simulink model "three_level_svpwm"  (R2013a)
settings: Solver=ode45  StartTime=0.0  StopTime=1  MaxStep=1e-3  RelTol=1e-3
libraries: powerlib x13, simulink x8, commutil2 x4, powerlib_meascontrol x3
settings Model: Creator=HXXXIA001  LastModifiedBy=HXXXIA001

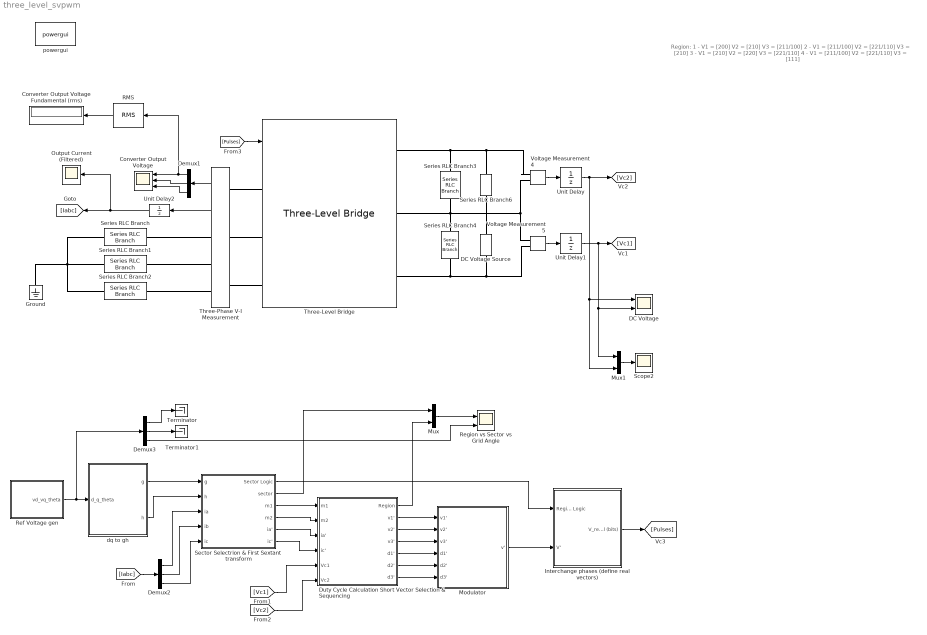
== system three_level_svpwm ==
  note: Region:
      | 1 - V1 = [200]	   V2 = [210]   V3 = [211/100]
      | 2 - V1 = [211/100]   V2 = [221/110]   V3 = [210]
      | 3 - V1 = [210]   V2 = [220]   V3 = [221/110]
      | 4 - V1 = [211/100]   V2 = [221/110]   V3 = [111]
  Converter Output Voltage : Scope  NumInputPorts=3
      settings: YMin=-120~-120~-120  YMax=120~120~120  SaveName=Vph
  Converter Output Voltage Fundamental (rms) : Display
  DC Voltage : Scope  NumInputPorts=2
      settings: YMin=59.65~59.725  YMax=60.3~60.275
  DC Voltage Source : powerlib/Electrical Sources/DC Voltage Source  Amplitude=120  Measurements=None
  Demux1 : Demux  Outputs=3
  Demux2 : Demux  Outputs=3
  Demux3 : Demux  Outputs=3
  Duty Cycle Calculation Short Vector Selection & Sequencing : Subsystem
  Ground : powerlib/Elements/Ground  LConnTagsString=a
  Interchange phases (define real vectors) : Subsystem
  Modulator : Subsystem  mask{Tm=5e-5, Ts=5e-6}
      mask prompts: Tm "Converter Modulation Period (s)"; Ts "Clock Sampling Period (s)"
  Mux : Mux  Inputs=2
  Mux1 : Mux  Inputs=2
  Output Current (Filtered) : Scope
      settings: YMin=-80  YMax=80  SaveName=Iph
  RMS : powerlib_meascontrol/Measurements/RMS  TrueRMS=on  Freq=50  RMSInit=0  Ts=5e-5
  Ref Voltage gen : Subsystem  mask{m=0.8, f=50}
      mask prompts: m "Modulation Index ( 0<m<1 )"; f "Fundamental Frequency (Hz)"
  Region vs Sector vs Grid Angle : Scope  NumInputPorts=2
      settings: YMin=-5~-5  YMax=5~5  SaveName=ScopeData3
  Scope2 : Scope
      settings: SaveName=ScopeData2
  Sector Selectrion & First Sextant transform : Subsystem
  Series RLC Branch : powerlib/Elements/Series RLC Branch  LConnTagsString=__new0  RConnTagsString=__new0  BranchType=RL  Resistance=10  Inductance=4e-3  SetiL0=off  InitialCurrent=0  Capacitance=1e-6  Setx0=off  InitialVoltage=0  Measurements=None
  Series RLC Branch1 : powerlib/Elements/Series RLC Branch  LConnTagsString=__new0  RConnTagsString=__new0  BranchType=RL  Resistance=10  Inductance=4e-3  SetiL0=off  InitialCurrent=0  Capacitance=1e-6  Setx0=off  InitialVoltage=0  Measurements=None
  Series RLC Branch2 : powerlib/Elements/Series RLC Branch  LConnTagsString=__new0  RConnTagsString=__new0  BranchType=RL  Resistance=10  Inductance=4e-3  SetiL0=off  InitialCurrent=0  Capacitance=1e-6  Setx0=off  InitialVoltage=0  Measurements=None
  Series RLC Branch3 : powerlib/Elements/Series RLC Branch  LConnTagsString=__new0  RConnTagsString=__new0  BranchType=C  Resistance=0.0001  Inductance=1e-3  SetiL0=off  InitialCurrent=0  Capacitance=4700e-6  Setx0=on  InitialVoltage=60  Measurements=None
  Series RLC Branch4 : powerlib/Elements/Series RLC Branch  LConnTagsString=__new0  RConnTagsString=__new0  BranchType=C  Resistance=0.0001  Inductance=1e-3  SetiL0=off  InitialCurrent=0  Capacitance=4700e-6  Setx0=on  InitialVoltage=60  Measurements=None
  Series RLC Branch6 : powerlib/Elements/Series RLC Branch  LConnTagsString=__new0  RConnTagsString=__new0  BranchType=R  Resistance=1e-3  Inductance=1e-3  SetiL0=off  InitialCurrent=0  Capacitance=4700e-6  Setx0=off  InitialVoltage=0  Measurements=None
  Terminator : Terminator
  Terminator1 : Terminator
  Three-Level Bridge : powerlib/Power Electronics/Three-Level Bridge  Arms=3  SnubberResistance=1e5  SbubberCapacitance=inf  Device=IGBT / Diodes  Ron=1e-3  ForwardVoltages="[  0  0  ]"  Measurements=None
  Three-Phase V-I Measurement : powerlib/Measurements/Three-Phase V-I Measurement  VoltageMeasurement=phase-to-ground  SetLabelV=off  LabelV=Vabc  Vpu=off  VpuLL=off  CurrentMeasurement=yes  SetLabelI=off  LabelI=Iabc  Ipu=off  Pbase=100e6  Vbase=500e3  OutputType=Complex  PhasorSimulation=off  PSBequivalent=0
  Unit Delay : UnitDelay  SampleTime=-1
  Unit Delay1 : UnitDelay  SampleTime=-1
  Unit Delay2 : UnitDelay  SampleTime=-1
  Voltage Measurement4 : powerlib/Measurements/Voltage Measurement  PhasorSimulation=off  OutputType=Complex  PSBequivalent=0
  Voltage Measurement5 : powerlib/Measurements/Voltage Measurement  PhasorSimulation=off  OutputType=Complex  PSBequivalent=0
  dq to gh : Subsystem
  powergui : powerlib/powergui  Priority=1  SimulationMode=Discrete  SolverType=Tustin  SampleTime=5e-6  frequency=60  SPID=off  DisableSnubberDevices=off  DisableRonSwitches=off  DisableVfSwitches=off  SwTol=0  Interpol=off  DisplayEquations=off  frequencyindice=0  Pbase=100e6  ErrMax=1e-4  Iterations=50  UnitsV=kV  UnitsW=MW  FunctionMessages=off  echomessages=off  HookPort=off  EnableUseOfTLC=off  x0status=blocks  RestoreLinks=warning  ResistiveCurrentMeasurement=off  Frange=[0:2:500]  Ylog=off  Xlog=on  ShowGrid=off  save=off  variable=ZData  structure=Iph  ZoomFFT=off  StartTime=0.0  cycles=10  DisplayStyle=1  fundamental=50  FreqAxis=off  MaxFrequency=2000  frequencyindicesteady=1  RmsSteady=1  display=off  Ts=0  methode=off
  wires:
  Ref Voltage gen/1(vd_vq_theta) -> Demux3/1, dq to gh/1(d_q_theta)
  Sector Selectrion & First Sextant transform/3(m1) -> Duty Cycle Calculation Short Vector Selection & Sequencing/1(m1)
  Sector Selectrion & First Sextant transform/4(m2) -> Duty Cycle Calculation Short Vector Selection & Sequencing/2(m2)
  Sector Selectrion & First Sextant transform/2(sector) -> Mux/1
  Mux/1 -> Region vs Sector vs Grid Angle/1
  Duty Cycle Calculation Short Vector Selection & Sequencing/1(Region) -> Mux/2
  dq to gh/1(g) -> Sector Selectrion & First Sextant transform/1(g)
  dq to gh/2(h) -> Sector Selectrion & First Sextant transform/2(h)
  Sector Selectrion & First Sextant transform/5(ia') -> Duty Cycle Calculation Short Vector Selection & Sequencing/3(ia')
  Sector Selectrion & First Sextant transform/6(ic') -> Duty Cycle Calculation Short Vector Selection & Sequencing/4(ic')
  Duty Cycle Calculation Short Vector Selection & Sequencing/2(v1') -> Modulator/1(v1')
  Duty Cycle Calculation Short Vector Selection & Sequencing/3(v2') -> Modulator/2(v2')
  Duty Cycle Calculation Short Vector Selection & Sequencing/4(v3') -> Modulator/3(v3')
  Duty Cycle Calculation Short Vector Selection & Sequencing/5(d1') -> Modulator/4(d1')
  Duty Cycle Calculation Short Vector Selection & Sequencing/6(d2') -> Modulator/5(d2')
  Duty Cycle Calculation Short Vector Selection & Sequencing/7(d3') -> Modulator/6(d3')
  Sector Selectrion & First Sextant transform/1(Sector Logic) -> Interchange phases (define real vectors)/1(Region Logic)
  Modulator/1(v') -> Interchange phases (define real vectors)/2(V')
  Three-Phase V-I Measurement/1 -> Demux1/1
  Demux1/1 -> Converter Output Voltage/1, RMS/1
  Demux1/2 -> Converter Output Voltage/2
  Demux1/3 -> Converter Output Voltage/3
  Voltage Measurement4/1 -> Unit Delay/1
  Unit Delay/1 -> Mux1/2, DC Voltage/1, [Vc2]
  Voltage Measurement5/1 -> Unit Delay1/1
  Unit Delay1/1 -> Mux1/1, DC Voltage/2, [Vc1]
  [Iabc] -> Demux2/1
  Demux2/1 -> Sector Selectrion & First Sextant transform/3(ia)
  Demux2/2 -> Sector Selectrion & First Sextant transform/4(ib)
  Demux2/3 -> Sector Selectrion & First Sextant transform/5(ic)
  [Vc1] -> Duty Cycle Calculation Short Vector Selection & Sequencing/5(Vc1)
  [Vc2] -> Duty Cycle Calculation Short Vector Selection & Sequencing/6(Vc2)
  Three-Phase V-I Measurement/2 -> Unit Delay2/1
  Unit Delay2/1 -> Output Current (Filtered)/1, [Iabc]
  Mux1/1 -> Scope2/1
  RMS/1 -> Converter Output Voltage Fundamental (rms)/1
  Demux3/1 -> Terminator/1
  Demux3/2 -> Terminator1/1
  Demux3/3 -> Region vs Sector vs Grid Angle/2
  Interchange phases (define real vectors)/1(V_real (bits)) -> [Pulses]
  [Pulses] -> Three-Level Bridge/1
  connections:
  Voltage Measurement4/LConn1 -- Series RLC Branch6/LConn1 -- Three-Level Bridge/RConn1 -- Series RLC Branch3/LConn1
  Voltage Measurement5/LConn2 -- Three-Level Bridge/RConn3 -- Series RLC Branch4/RConn1 -- DC Voltage Source/LConn1
  Series RLC Branch/RConn1 -- Ground/LConn1 -- Series RLC Branch2/RConn1 -- Series RLC Branch1/RConn1
  Three-Phase V-I Measurement/LConn1 -- Three-Level Bridge/LConn1
  Three-Phase V-I Measurement/LConn2 -- Three-Level Bridge/LConn2
  Three-Phase V-I Measurement/LConn3 -- Three-Level Bridge/LConn3
  Series RLC Branch/LConn1 -- Three-Phase V-I Measurement/RConn1
  Series RLC Branch1/LConn1 -- Three-Phase V-I Measurement/RConn2
  Series RLC Branch2/LConn1 -- Three-Phase V-I Measurement/RConn3
  Voltage Measurement4/LConn2 -- Three-Level Bridge/RConn2 -- Series RLC Branch4/LConn1 -- Series RLC Branch3/RConn1 -- Voltage Measurement5/LConn1
  Series RLC Branch6/RConn1 -- DC Voltage Source/RConn1

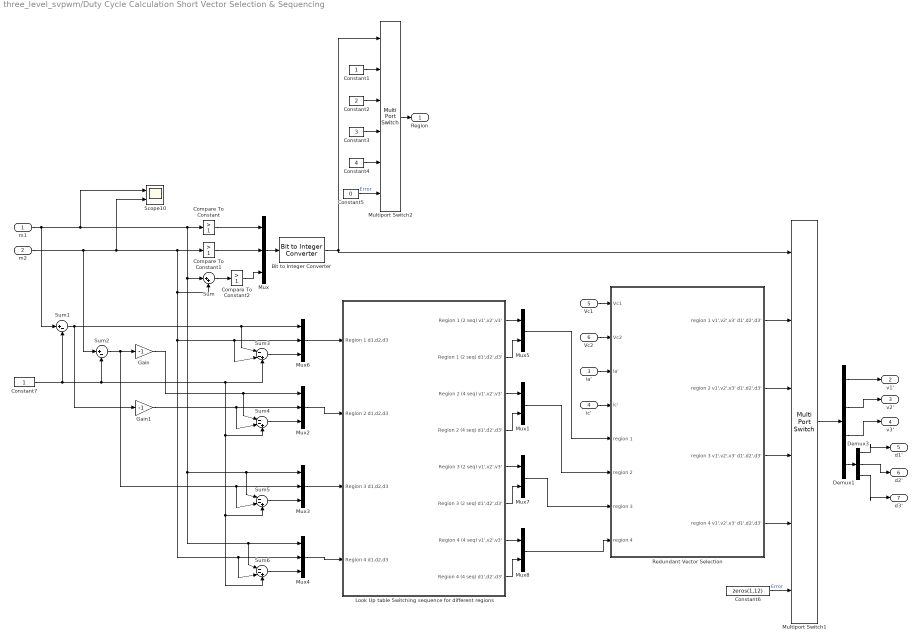
== system three_level_svpwm/Duty Cycle Calculation Short Vector Selection & Sequencing ==
  m1 : Inport
  m2 : Inport  Port=2
  ia' : Inport  Port=3
  ic' : Inport  Port=4
  Vc1 : Inport  Port=5
  Vc2 : Inport  Port=6
  Bit to Integer Converter : commutil2/Bit to Integer Converter  nbits=3  bitOrder=MSB first  signedOutputValues=Unsigned  outDtype=Inherit via internal rule  outDtypeSigned=Inherit via internal rule
  Compare To Constant : simulink/Logic and Bit Operations/Compare To Constant  relop=>  const=1  OutDataTypeStr=boolean
  Compare To Constant1 : simulink/Logic and Bit Operations/Compare To Constant  relop=>  const=1  OutDataTypeStr=boolean
  Compare To Constant2 : simulink/Logic and Bit Operations/Compare To Constant  relop=>  const=1  OutDataTypeStr=boolean
  Constant1 : Constant
  Constant2 : Constant  Value=2
  Constant3 : Constant  Value=3
  Constant4 : Constant  Value=4
  Constant5 : Constant  Value=0
  Constant6 : Constant  Value=zeros(1,12)
  Constant7 : Constant
  Demux1 : Demux
  Demux3 : Demux  Outputs=3
  Gain : Gain  Gain=-1
  Gain1 : Gain  Gain=-1
  Look Up table Switching sequence for different regions : Subsystem
  Multiport Switch1 : MultiPortSwitch  DataPortOrder=Specify indices  Inputs=6  DataPortIndices={5,1,3,0,[2,4,6,7]}
  Multiport Switch2 : MultiPortSwitch  DataPortOrder=Specify indices  Inputs=6  DataPortIndices={5,1,3,0,[2,4,6,7]}
  Mux{,2..4,6} (5 alike) : Mux  Inputs=3
  Mux{1,5,7..8} (4 alike) : Mux  Inputs=2
  Redundant Vector Selection : Subsystem
  Scope10 : Scope  NumInputPorts=2
      settings: YMin=0~-5  YMax=1.75~5  SaveName=ScopeData17
  Sum : Sum  Inputs=|++
  Sum1 : Sum  Inputs=|+-
  Sum2 : Sum  Inputs=|+-
  Sum{3..6} (4 alike) : Sum  Inputs=|--+
  Region : Outport
  v1' : Outport  Port=2
  v2' : Outport  Port=3
  v3' : Outport  Port=4
  d1' : Outport  Port=5
  d2' : Outport  Port=6
  d3' : Outport  Port=7
  wires:
  Compare To Constant2/1 -> Mux/3
  Sum/1 -> Compare To Constant2/1
  m1/1 -> Scope10/1, Sum6/1, Mux4/1, Sum5/1, Mux3/1, Sum/1, Compare To Constant/1, Sum1/1
  m2/1 -> Scope10/2, Sum6/2, Mux4/2, Mux6/2, Sum3/2, Sum/2, Compare To Constant1/1, Sum2/1
  Constant4/1 -> Multiport Switch2/5
  Constant5/1 -> Multiport Switch2/6  "Error"
  Multiport Switch2/1 -> Region/1
  Constant6/1 -> Multiport Switch1/6  "Error"
  Compare To Constant/1 -> Mux/1
  Constant3/1 -> Multiport Switch2/4
  Constant1/1 -> Multiport Switch2/2
  Constant2/1 -> Multiport Switch2/3
  Bit to Integer Converter/1 -> Multiport Switch1/1, Multiport Switch2/1
  Compare To Constant1/1 -> Mux/2
  Mux/1 -> Bit to Integer Converter/1
  Constant7/1 -> Sum1/2, Sum6/3, Sum5/3, Sum4/3, Sum3/3, Sum2/2
  Sum1/1 -> Gain1/1, Mux6/1, Sum3/1
  Sum3/1 -> Mux6/3
  Gain/1 -> Sum4/1, Mux2/1
  Sum2/1 -> Sum5/2, Mux3/2, Gain/1
  Gain1/1 -> Sum4/2, Mux2/2
  Sum4/1 -> Mux2/3
  Sum5/1 -> Mux3/3
  Sum6/1 -> Mux4/3
  Vc1/1 -> Redundant Vector Selection/1(Vc1)
  Vc2/1 -> Redundant Vector Selection/2(Vc2)
  ia'/1 -> Redundant Vector Selection/3(ia')
  ic'/1 -> Redundant Vector Selection/4(ic')
  Mux6/1 -> Look Up table Switching sequence for different regions/1(Region 1 d1,d2,d3)
  Mux2/1 -> Look Up table Switching sequence for different regions/2(Region 2 d1,d2,d3)
  Mux3/1 -> Look Up table Switching sequence for different regions/3(Region 3 d1,d2,d3)
  Mux4/1 -> Look Up table Switching sequence for different regions/4(Region 4 d1,d2,d3)
  Look Up table Switching sequence for different regions/1(Region 1 (2 seq) v1',v2',v3') -> Mux5/1
  Look Up table Switching sequence for different regions/2(Region 1 (2 seq) d1',d2',d3') -> Mux5/2
  Look Up table Switching sequence for different regions/3(Region 2 (4 seq) v1',v2',v3') -> Mux1/1
  Look Up table Switching sequence for different regions/4(Region 2 (4 seq) d1',d2',d3') -> Mux1/2
  Look Up table Switching sequence for different regions/5(Region 3 (2 seq) v1',v2',v3') -> Mux7/1
  Look Up table Switching sequence for different regions/6(Region 3 (2 seq) d1',d2',d3') -> Mux7/2
  Look Up table Switching sequence for different regions/7(Region 4 (4 seq) v1',v2',v3') -> Mux8/1
  Look Up table Switching sequence for different regions/8(Region 4 (4 seq) d1',d2',d3') -> Mux8/2
  Mux5/1 -> Redundant Vector Selection/5(region 1)
  Mux1/1 -> Redundant Vector Selection/6(region 2)
  Mux7/1 -> Redundant Vector Selection/7(region 3)
  Mux8/1 -> Redundant Vector Selection/8(region 4)
  Redundant Vector Selection/1(region 1 v1',v2',v3' d1',d2',d3') -> Multiport Switch1/2
  Redundant Vector Selection/2(region 2 v1',v2',v3' d1',d2',d3') -> Multiport Switch1/3
  Redundant Vector Selection/3(region 3 v1',v2',v3' d1',d2',d3') -> Multiport Switch1/4
  Redundant Vector Selection/4(region 4 v1',v2',v3' d1',d2',d3') -> Multiport Switch1/5
  Multiport Switch1/1 -> Demux1/1
  Demux1/4 -> Demux3/1
  Demux1/1 -> v1'/1
  Demux1/2 -> v2'/1
  Demux1/3 -> v3'/1
  Demux3/1 -> d1'/1
  Demux3/2 -> d2'/1
  Demux3/3 -> d3'/1

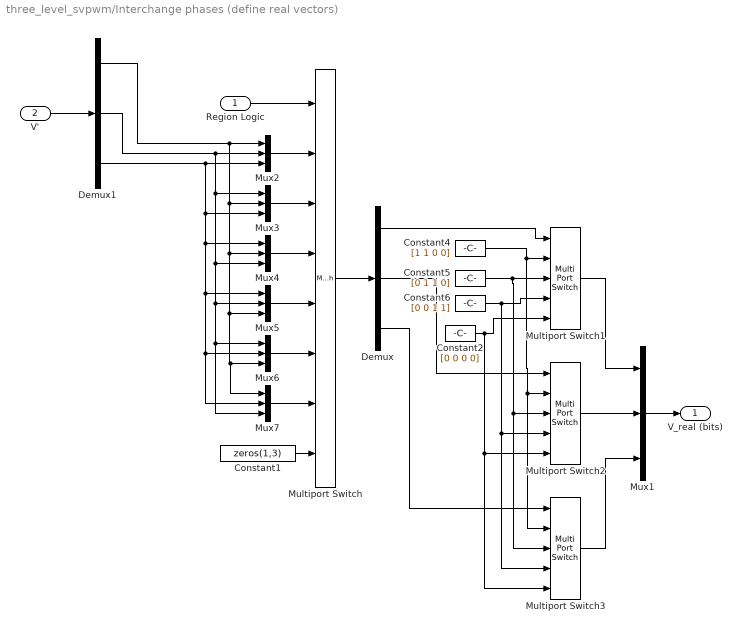
== system three_level_svpwm/Interchange phases (define real vectors) ==
  Region Logic : Inport
  V' : Inport  Port=2
  Constant1 : Constant  Value=zeros(1,3)
  Constant2 : Constant  Value=[0 0 0 0]
  Constant4 : Constant  Value=[1 1 0 0]
  Constant5 : Constant  Value=[0 1 1 0]
  Constant6 : Constant  Value=[0 0 1 1]
  Demux : Demux  Outputs=3
  Demux1 : Demux  Outputs=3
  Multiport Switch : MultiPortSwitch  DataPortOrder=Specify indices  Inputs=6  DataPortIndices={7,3,2,0,4,5,[1,6]}
  Multiport Switch1 : MultiPortSwitch  DataPortOrder=Specify indices  Inputs=6  DataPortIndices={2,1,0}  DataPortForDefault=Additional data port
  Multiport Switch2 : MultiPortSwitch  DataPortOrder=Specify indices  Inputs=6  DataPortIndices={2,1,0}  DataPortForDefault=Additional data port
  Multiport Switch3 : MultiPortSwitch  DataPortOrder=Specify indices  Inputs=6  DataPortIndices={2,1,0}  DataPortForDefault=Additional data port
  Mux{1..7} (7 alike) : Mux  Inputs=3
  V_real (bits) : Outport
  wires:
  Constant1/1 -> Multiport Switch/8
  Mux5/1 -> Multiport Switch/5
  V'/1 -> Demux1/1
  Mux4/1 -> Multiport Switch/4
  Demux1/2 -> Mux7/3, Mux6/1, Mux5/2, Mux4/3, Mux3/1, Mux2/2
  Demux1/1 -> Mux7/1, Mux6/3, Mux5/3, Mux4/2, Mux3/2, Mux2/1
  Demux1/3 -> Mux6/2, Mux7/2, Mux5/1, Mux4/1, Mux3/3, Mux2/3
  Mux6/1 -> Multiport Switch/6
  Mux7/1 -> Multiport Switch/7
  Mux2/1 -> Multiport Switch/2
  Region Logic/1 -> Multiport Switch/1
  Mux3/1 -> Multiport Switch/3
  Multiport Switch3/1 -> Mux1/3
  Multiport Switch2/1 -> Mux1/2
  Multiport Switch1/1 -> Mux1/1
  Constant4/1 -> Multiport Switch3/2, Multiport Switch2/2, Multiport Switch1/2
  Constant5/1 -> Multiport Switch3/3, Multiport Switch2/3, Multiport Switch1/3
  Constant6/1 -> Multiport Switch3/4, Multiport Switch2/4, Multiport Switch1/4
  Demux/2 -> Multiport Switch2/1
  Demux/3 -> Multiport Switch3/1
  Multiport Switch/1 -> Demux/1
  Demux/1 -> Multiport Switch1/1
  Mux1/1 -> V_real (bits)/1
  Constant2/1 -> Multiport Switch1/5, Multiport Switch3/5, Multiport Switch2/5

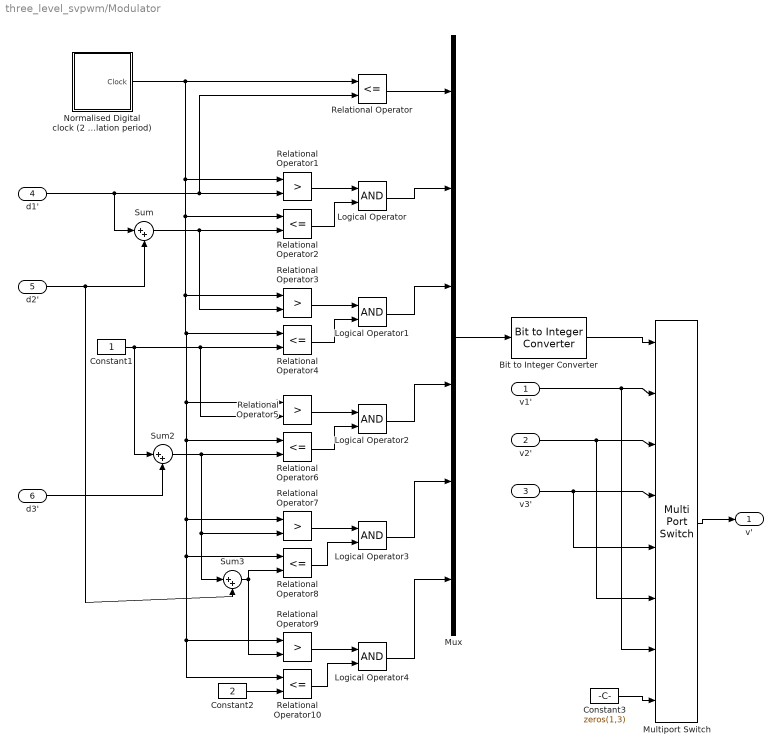
== system three_level_svpwm/Modulator ==
  v1' : Inport
  v2' : Inport  Port=2
  v3' : Inport  Port=3
  d1' : Inport  Port=4
  d2' : Inport  Port=5
  d3' : Inport  Port=6
  Bit to Integer Converter : commutil2/Bit to Integer Converter  nbits=6  bitOrder=MSB first  signedOutputValues=Unsigned  outDtype=Inherit via internal rule  outDtypeSigned=Inherit via internal rule
  Constant1 : Constant
  Constant2 : Constant  Value=2
  Constant3 : Constant  Value=zeros(1,3)
  Logical Operator{,1..4} (5 alike) : Logic  AllPortsSameDT=off  OutDataTypeStr=boolean
  Multiport Switch : MultiPortSwitch  DataPortOrder=Specify indices  DataPortIndices={32,16,8,4,2,1,[0,3,5:7,9:15,17:31,33:64]}
  Mux : Mux  Inputs=6
  Normalised Digital clock (2 Modulation period) : Subsystem  mask{Tm=Tm, Ts=Ts}
      mask prompts: Tm "Converter Modulation Period (s)"; Ts "Clock Sampling Period (s)"
      mask help:
      | Make Sure Clock Sampling is much faster than converter modulation period
      | for accurate calculations.
      |
      | Note: Higher Sampling rate will make simulation slow, however, it can be
      | easily implemented with FPGA.
  Relational Operator{,2,4,6,8,10} (6 alike) : RelationalOperator  Operator=<=  OutDataTypeStr=boolean
  Relational Operator{1,3,5,7,9} (5 alike) : RelationalOperator  Operator=>  OutDataTypeStr=boolean
  Sum : Sum  Inputs=|++
  Sum2 : Sum  Inputs=|++
  Sum3 : Sum  Inputs=|++
  v' : Outport
  wires:
  Sum/1 -> Relational Operator3/2, Relational Operator2/2
  d1'/1 -> Sum/1, Relational Operator/2, Relational Operator1/2
  d2'/1 -> Sum/2, Sum3/2
  Constant1/1 -> Sum2/1, Relational Operator5/2, Relational Operator4/2
  Normalised Digital clock (2 Modulation period)/1(Clock) -> Relational Operator9/1, Relational Operator10/1, Relational Operator8/1, Relational Operator7/1, Relational Operator6/1, Relational Operator5/1, Relational Operator4/1, Relational Operator3/1, Relational Operator2/1, Relational Operator1/1, Relational Operator/1
  Relational Operator9/1 -> Logical Operator4/1
  Relational Operator1/1 -> Logical Operator/1
  d3'/1 -> Sum2/2
  Sum2/1 -> Sum3/1, Relational Operator7/2, Relational Operator6/2
  Sum3/1 -> Relational Operator9/2, Relational Operator8/2
  Relational Operator8/1 -> Logical Operator3/2
  Relational Operator7/1 -> Logical Operator3/1
  Relational Operator6/1 -> Logical Operator2/2
  Constant2/1 -> Relational Operator10/2
  Relational Operator4/1 -> Logical Operator1/2
  Relational Operator10/1 -> Logical Operator4/2
  Relational Operator2/1 -> Logical Operator/2
  Relational Operator5/1 -> Logical Operator2/1
  Relational Operator3/1 -> Logical Operator1/1
  Relational Operator/1 -> Mux/1
  Logical Operator/1 -> Mux/2
  Logical Operator1/1 -> Mux/3
  Logical Operator2/1 -> Mux/4
  Logical Operator3/1 -> Mux/5
  Logical Operator4/1 -> Mux/6
  Mux/1 -> Bit to Integer Converter/1
  Bit to Integer Converter/1 -> Multiport Switch/1
  v1'/1 -> Multiport Switch/7, Multiport Switch/2
  v2'/1 -> Multiport Switch/6, Multiport Switch/3
  v3'/1 -> Multiport Switch/5, Multiport Switch/4
  Constant3/1 -> Multiport Switch/8
  Multiport Switch/1 -> v'/1

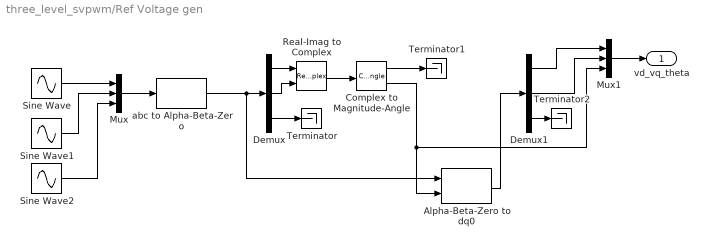
== system three_level_svpwm/Ref Voltage gen ==
  Alpha-Beta-Zero to dq0 : powerlib_meascontrol/Transformations/Alpha-Beta-Zero to dq0  Alignment=Aligned with phase A axis
  Complex to Magnitude-Angle : ComplexToMagnitudeAngle
  Demux : Demux  Outputs=3
  Demux1 : Demux  Outputs=3
  Mux : Mux  Inputs=3
  Mux1 : Mux  Inputs=3
  Real-Imag to Complex : RealImagToComplex
  Sine Wave : Sin  Amplitude=m*sqrt(3)  Frequency=2*pi*f  SampleTime=0
  Sine Wave1 : Sin  Amplitude=m*sqrt(3)  Frequency=2*pi*f  Phase=-2*pi/3  SampleTime=0
  Sine Wave2 : Sin  Amplitude=m*sqrt(3)  Frequency=2*pi*f  Phase=2*pi/3  SampleTime=0
  Terminator : Terminator
  Terminator1 : Terminator
  Terminator2 : Terminator
  abc to Alpha-Beta-Zero : powerlib_meascontrol/Transformations/abc to Alpha-Beta-Zero
  vd_vq_theta : Outport
  wires:
  Demux1/2 -> Mux1/2
  Demux1/3 -> Terminator2/1
  Demux1/1 -> Mux1/1
  Demux/3 -> Terminator/1
  Demux/2 -> Real-Imag to Complex/2
  Demux/1 -> Real-Imag to Complex/1
  Real-Imag to Complex/1 -> Complex to Magnitude-Angle/1
  Complex to Magnitude-Angle/1 -> Terminator1/1
  abc to Alpha-Beta-Zero/1 -> Alpha-Beta-Zero to dq0/1, Demux/1
  Alpha-Beta-Zero to dq0/1 -> Demux1/1
  Sine Wave2/1 -> Mux/3
  Complex to Magnitude-Angle/2 -> Mux1/3, Alpha-Beta-Zero to dq0/2
  Sine Wave1/1 -> Mux/2
  Mux/1 -> abc to Alpha-Beta-Zero/1
  Sine Wave/1 -> Mux/1
  Mux1/1 -> vd_vq_theta/1

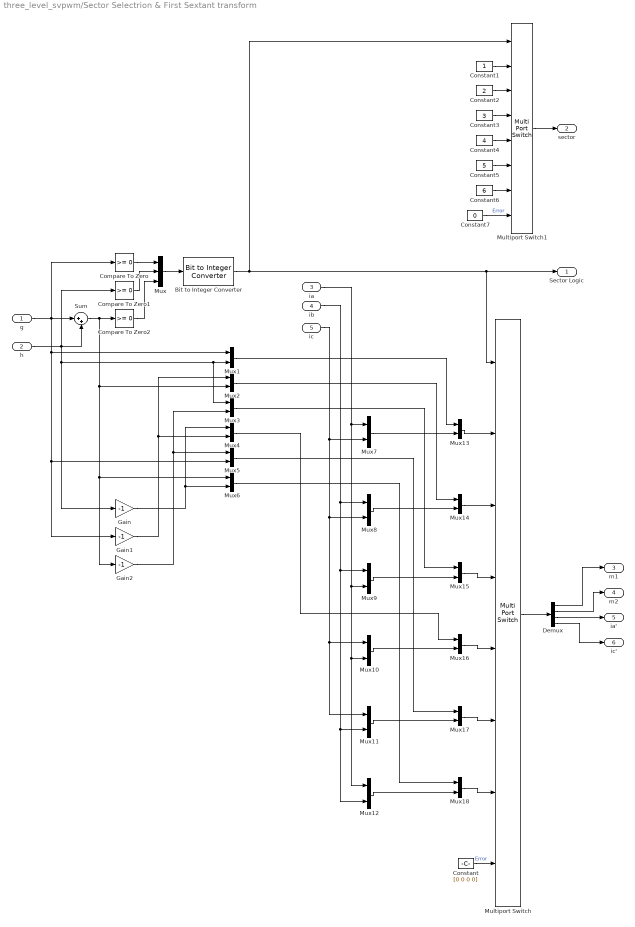
== system three_level_svpwm/Sector Selectrion & First Sextant transform ==
  g : Inport
  h : Inport  Port=2
  ia : Inport  Port=3
  ib : Inport  Port=4
  ic : Inport  Port=5
  Bit to Integer Converter : commutil2/Bit to Integer Converter  nbits=3  bitOrder=MSB first  signedOutputValues=Unsigned  outDtype=Inherit via internal rule  outDtypeSigned=Inherit via internal rule
  Compare To Zero : simulink/Logic and Bit Operations/Compare To Zero  relop=>=  OutDataTypeStr=boolean
  Compare To Zero1 : simulink/Logic and Bit Operations/Compare To Zero  relop=>=  OutDataTypeStr=boolean
  Compare To Zero2 : simulink/Logic and Bit Operations/Compare To Zero  relop=>=  OutDataTypeStr=boolean
  Constant : Constant  Value=[0 0 0 0]
  Constant1 : Constant
  Constant2 : Constant  Value=2
  Constant3 : Constant  Value=3
  Constant4 : Constant  Value=4
  Constant5 : Constant  Value=5
  Constant6 : Constant  Value=6
  Constant7 : Constant  Value=0
  Demux : Demux
  Gain : Gain  Gain=-1
  Gain1 : Gain  Gain=-1
  Gain2 : Gain  Gain=-1
  Multiport Switch : MultiPortSwitch  DataPortOrder=Specify indices  Inputs=6  DataPortIndices={7,3,2,0,4,5,[1,6]}
  Multiport Switch1 : MultiPortSwitch  DataPortOrder=Specify indices  Inputs=6  DataPortIndices={7,3,2,0,4,5,[1,6]}
  Mux : Mux  Inputs=3
  Mux{1..18} (18 alike) : Mux  Inputs=2
  Sum : Sum  Inputs=|++
  Sector Logic : Outport
  sector : Outport  Port=2
  m1 : Outport  Port=3
  m2 : Outport  Port=4
  ia' : Outport  Port=5
  ic' : Outport  Port=6
  wires:
  Compare To Zero1/1 -> Mux/2
  Compare To Zero/1 -> Mux/1
  Mux/1 -> Bit to Integer Converter/1
  Compare To Zero2/1 -> Mux/3
  Sum/1 -> Mux6/1, Gain2/1, Mux2/2, Compare To Zero2/1
  g/1 -> Mux5/2, Gain1/1, Mux1/1, Compare To Zero/1, Sum/1
  Bit to Integer Converter/1 -> Multiport Switch1/1, Sector Logic/1, Multiport Switch/1
  Gain1/1 -> Mux4/2, Mux2/1
  h/1 -> Sum/2, Gain/1, Mux3/1, Mux1/2, Compare To Zero1/1
  Gain2/1 -> Mux5/1, Mux3/2
  Gain/1 -> Mux6/2, Mux4/1
  Constant/1 -> Multiport Switch/8  "Error"
  Constant1/1 -> Multiport Switch1/2
  Constant2/1 -> Multiport Switch1/3
  Constant3/1 -> Multiport Switch1/4
  Constant4/1 -> Multiport Switch1/5
  Constant5/1 -> Multiport Switch1/6
  Constant6/1 -> Multiport Switch1/7
  Constant7/1 -> Multiport Switch1/8  "Error"
  Multiport Switch1/1 -> sector/1
  Multiport Switch/1 -> Demux/1
  Demux/1 -> m1/1
  Demux/2 -> m2/1
  Mux7/1 -> Mux13/2
  Mux1/1 -> Mux13/1
  Mux8/1 -> Mux14/2
  Mux2/1 -> Mux14/1
  Mux9/1 -> Mux15/2
  Mux3/1 -> Mux15/1
  Mux10/1 -> Mux16/2
  Mux4/1 -> Mux16/1
  Mux11/1 -> Mux17/2
  Mux5/1 -> Mux17/1
  Mux12/1 -> Mux18/2
  Mux6/1 -> Mux18/1
  Mux13/1 -> Multiport Switch/2
  Mux14/1 -> Multiport Switch/3
  Mux15/1 -> Multiport Switch/4
  Mux16/1 -> Multiport Switch/5
  Mux17/1 -> Multiport Switch/6
  Mux18/1 -> Multiport Switch/7
  ia/1 -> Mux12/1, Mux10/2, Mux9/2, Mux7/1
  ic/1 -> Mux11/1, Mux10/1, Mux8/2, Mux7/2
  ib/1 -> Mux8/1, Mux11/2, Mux12/2, Mux9/1
  Demux/3 -> ia'/1
  Demux/4 -> ic'/1

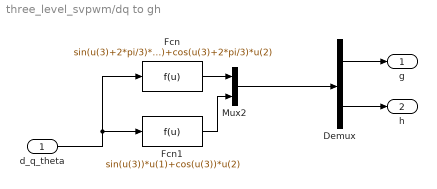
== system three_level_svpwm/dq to gh ==
  d_q_theta : Inport
  Demux : Demux  Outputs=2
  Fcn : Fcn  Expr=sin(u(3)+2*pi/3)*u(1)+cos(u(3)+2*pi/3)*u(2)
  Fcn1 : Fcn  Expr=sin(u(3))*u(1)+cos(u(3))*u(2)
  Mux2 : Mux  Inputs=2
  g : Outport
  h : Outport  Port=2
  wires:
  Fcn/1 -> Mux2/1
  d_q_theta/1 -> Fcn1/1, Fcn/1
  Fcn1/1 -> Mux2/2
  Mux2/1 -> Demux/1
  Demux/1 -> g/1
  Demux/2 -> h/1

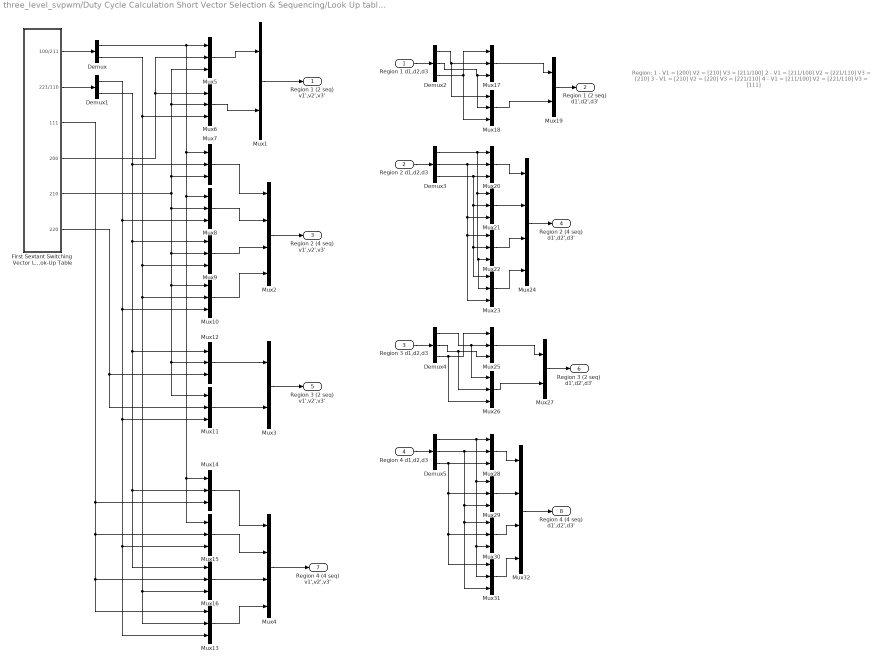
== system three_level_svpwm/Duty Cycle Calculation Short Vector Selection & Sequencing/Look Up table Switching sequence for different regions ==
  note: Region:
      | 1 - V1 = [200]	   V2 = [210]   V3 = [211/100]
      | 2 - V1 = [211/100]   V2 = [221/110]   V3 = [210]
      | 3 - V1 = [210]   V2 = [220]   V3 = [221/110]
      | 4 - V1 = [211/100]   V2 = [221/110]   V3 = [111]
  Region 1 d1,d2,d3 : Inport
  Region 2 d1,d2,d3 : Inport  Port=2
  Region 3 d1,d2,d3 : Inport  Port=3
  Region 4 d1,d2,d3 : Inport  Port=4
  Demux : Demux  Outputs=2
  Demux1 : Demux  Outputs=2
  Demux{2..5} (4 alike) : Demux  Outputs=3
  First Sextant Switching Vector Look-Up Table : Subsystem
  Mux{1,3,19,27} (4 alike) : Mux  Inputs=2
  Mux{5..18,20..23,25..26,28..31} (24 alike) : Mux  Inputs=3
  Mux{2,4,24,32} (4 alike) : Mux
  Region 1 (2 seq) v1',v2',v3' : Outport
  Region 1 (2 seq) d1',d2',d3' : Outport  Port=2
  Region 2 (4 seq) v1',v2',v3' : Outport  Port=3
  Region 2 (4 seq) d1',d2',d3' : Outport  Port=4
  Region 3 (2 seq) v1',v2',v3' : Outport  Port=5
  Region 3 (2 seq) d1',d2',d3' : Outport  Port=6
  Region 4 (4 seq) v1',v2',v3' : Outport  Port=7
  Region 4 (4 seq) d1',d2',d3' : Outport  Port=8
  wires:
  First Sextant Switching Vector Look-Up Table/2(221/110) -> Demux1/1
  First Sextant Switching Vector Look-Up Table/3(111) -> Mux13/1, Mux16/2, Mux15/2, Mux14/3
  Demux1/2 -> Mux16/1, Mux14/2, Mux12/1, Mux9/1, Mux7/2
  Demux/1 -> Mux15/1, Mux14/1, Mux8/1, Mux7/1, Mux5/1
  First Sextant Switching Vector Look-Up Table/1(100/211) -> Demux/1
  Demux/2 -> Mux6/3, Mux13/2, Mux16/3, Mux10/2, Mux9/3
  Mux5/1 -> Mux1/1
  Mux14/1 -> Mux4/1
  Mux15/1 -> Mux4/2
  Mux6/1 -> Mux1/2
  Mux16/1 -> Mux4/3
  Mux9/1 -> Mux2/3
  Mux13/1 -> Mux4/4
  Mux10/1 -> Mux2/4
  Mux12/1 -> Mux3/1
  Mux8/1 -> Mux2/2
  Demux1/1 -> Mux13/3, Mux15/3, Mux11/3, Mux10/3, Mux8/3
  Mux7/1 -> Mux2/1
  Mux11/1 -> Mux3/2
  First Sextant Switching Vector Look-Up Table/6(220) -> Mux11/2, Mux12/3
  First Sextant Switching Vector Look-Up Table/5(210) -> Mux7/3, Mux6/2, Mux5/3, Mux11/1, Mux12/2, Mux10/1, Mux9/2, Mux8/2
  First Sextant Switching Vector Look-Up Table/4(200) -> Mux6/1, Mux5/2
  Mux1/1 -> Region 1 (2 seq) v1',v2',v3'/1
  Mux2/1 -> Region 2 (4 seq) v1',v2',v3'/1
  Mux3/1 -> Region 3 (2 seq) v1',v2',v3'/1
  Mux4/1 -> Region 4 (4 seq) v1',v2',v3'/1
  Region 1 d1,d2,d3/1 -> Demux2/1
  Demux2/3 -> Mux18/3, Mux17/1
  Demux2/1 -> Mux18/1, Mux17/2
  Demux2/2 -> Mux18/2, Mux17/3
  Mux17/1 -> Mux19/1
  Mux18/1 -> Mux19/2
  Mux19/1 -> Region 1 (2 seq) d1',d2',d3'/1
  Region 2 d1,d2,d3/1 -> Demux3/1
  Demux3/1 -> Mux23/2, Mux22/3, Mux21/1, Mux20/1
  Demux3/2 -> Mux22/1, Mux23/3, Mux21/3, Mux20/2
  Demux3/3 -> Mux21/2, Mux22/2, Mux23/1, Mux20/3
  Mux20/1 -> Mux24/1
  Mux21/1 -> Mux24/2
  Mux22/1 -> Mux24/3
  Mux23/1 -> Mux24/4
  Mux24/1 -> Region 2 (4 seq) d1',d2',d3'/1
  Region 3 d1,d2,d3/1 -> Demux4/1
  Demux4/3 -> Mux26/3, Mux25/1
  Demux4/1 -> Mux25/2, Mux26/1
  Demux4/2 -> Mux25/3, Mux26/2
  Mux25/1 -> Mux27/1
  Mux26/1 -> Mux27/2
  Mux27/1 -> Region 3 (2 seq) d1',d2',d3'/1
  Region 4 d1,d2,d3/1 -> Demux5/1
  Demux5/1 -> Mux31/2, Mux30/3, Mux29/1, Mux28/1
  Demux5/2 -> Mux31/3, Mux30/1, Mux29/3, Mux28/2
  Demux5/3 -> Mux31/1, Mux30/2, Mux29/2, Mux28/3
  Mux28/1 -> Mux32/1
  Mux29/1 -> Mux32/2
  Mux30/1 -> Mux32/3
  Mux31/1 -> Mux32/4
  Mux32/1 -> Region 4 (4 seq) d1',d2',d3'/1

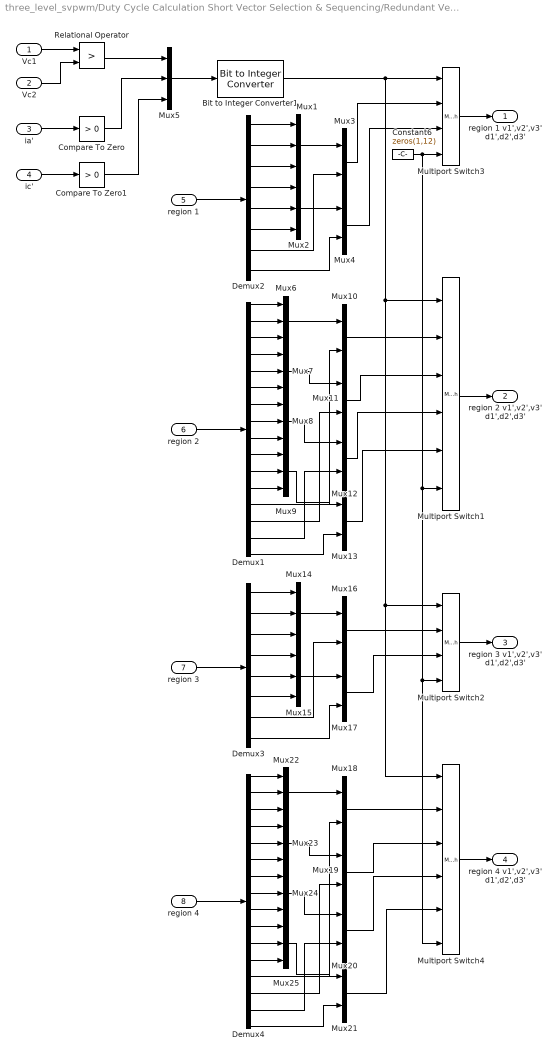
== system three_level_svpwm/Duty Cycle Calculation Short Vector Selection & Sequencing/Redundant Vector Selection ==
  Vc1 : Inport
  Vc2 : Inport  Port=2
  ia' : Inport  Port=3
  ic' : Inport  Port=4
  region 1 : Inport  Port=5
  region 2 : Inport  Port=6
  region 3 : Inport  Port=7
  region 4 : Inport  Port=8
  Bit to Integer Converter1 : commutil2/Bit to Integer Converter  nbits=3  bitOrder=MSB first  signedOutputValues=Unsigned  outDtype=Inherit via internal rule  outDtypeSigned=Inherit via internal rule
  Compare To Zero : simulink/Logic and Bit Operations/Compare To Zero  relop=>  OutDataTypeStr=boolean
  Compare To Zero1 : simulink/Logic and Bit Operations/Compare To Zero  relop=>  OutDataTypeStr=boolean
  Constant6 : Constant  Value=zeros(1,12)
  Demux1 : Demux  Outputs=16
  Demux2 : Demux  Outputs=8
  Demux3 : Demux  Outputs=8
  Demux4 : Demux  Outputs=16
  Multiport Switch1 : MultiPortSwitch  DataPortOrder=Specify indices  Inputs=6  DataPortIndices={[1,6],[0,7],[3,4],[2,5]}  DataPortForDefault=Additional data port
  Multiport Switch2 : MultiPortSwitch  DataPortOrder=Specify indices  Inputs=6  DataPortIndices={[1,3,4,6],[0,2,5,7]}  DataPortForDefault=Additional data port
  Multiport Switch3 : MultiPortSwitch  DataPortOrder=Specify indices  Inputs=6  DataPortIndices={[0,1,6,7],[2,3,4,5]}  DataPortForDefault=Additional data port
  Multiport Switch4 : MultiPortSwitch  DataPortOrder=Specify indices  Inputs=6  DataPortIndices={[1,6],[0,7],[3,4],[2,5]}  DataPortForDefault=Additional data port
  Mux{1..2,5..9,14..15,22..25} (13 alike) : Mux  Inputs=3
  Mux{3..4,10..13,16..21} (12 alike) : Mux  Inputs=2
  Relational Operator : RelationalOperator  Operator=>  OutDataTypeStr=boolean
  region 1 v1',v2',v3' d1',d2',d3' : Outport
  region 2 v1',v2',v3' d1',d2',d3' : Outport  Port=2
  region 3 v1',v2',v3' d1',d2',d3' : Outport  Port=3
  region 4 v1',v2',v3' d1',d2',d3' : Outport  Port=4
  wires:
  Vc1/1 -> Relational Operator/1
  ic'/1 -> Compare To Zero1/1
  Vc2/1 -> Relational Operator/2
  Bit to Integer Converter1/1 -> Multiport Switch4/1, Multiport Switch2/1, Multiport Switch1/1, Multiport Switch3/1
  ia'/1 -> Compare To Zero/1
  Compare To Zero/1 -> Mux5/2
  Mux5/1 -> Bit to Integer Converter1/1
  Relational Operator/1 -> Mux5/1
  Compare To Zero1/1 -> Mux5/3
  Multiport Switch3/1 -> region 1 v1',v2',v3' d1',d2',d3'/1
  Multiport Switch1/1 -> region 2 v1',v2',v3' d1',d2',d3'/1
  Multiport Switch2/1 -> region 3 v1',v2',v3' d1',d2',d3'/1
  Multiport Switch4/1 -> region 4 v1',v2',v3' d1',d2',d3'/1
  region 1/1 -> Demux2/1
  Demux2/1 -> Mux1/1
  Demux2/2 -> Mux1/2
  Demux2/3 -> Mux1/3
  Demux2/4 -> Mux2/1
  Demux2/5 -> Mux2/2
  Demux2/6 -> Mux2/3
  Mux1/1 -> Mux3/1
  Demux2/7 -> Mux3/2
  Mux3/1 -> Multiport Switch3/2
  Mux2/1 -> Mux4/1
  Demux2/8 -> Mux4/2
  Mux4/1 -> Multiport Switch3/3
  region 2/1 -> Demux1/1
  Demux1/1 -> Mux6/1
  Demux1/2 -> Mux6/2
  Demux1/3 -> Mux6/3
  Demux1/4 -> Mux7/1
  Demux1/5 -> Mux7/2
  Demux1/6 -> Mux7/3
  Demux1/7 -> Mux8/1
  Demux1/8 -> Mux8/2
  Demux1/9 -> Mux8/3
  Demux1/10 -> Mux9/1
  Demux1/11 -> Mux9/2
  Demux1/12 -> Mux9/3
  Mux6/1 -> Mux10/1
  Demux1/13 -> Mux10/2
  Mux7/1 -> Mux11/1
  Demux1/14 -> Mux11/2
  Mux8/1 -> Mux12/1
  Demux1/15 -> Mux12/2
  Mux9/1 -> Mux13/1
  Demux1/16 -> Mux13/2
  Mux10/1 -> Multiport Switch1/2
  Mux11/1 -> Multiport Switch1/3
  Mux12/1 -> Multiport Switch1/4
  Mux13/1 -> Multiport Switch1/5
  region 3/1 -> Demux3/1
  Demux3/1 -> Mux14/1
  Demux3/2 -> Mux14/2
  Demux3/3 -> Mux14/3
  Demux3/4 -> Mux15/1
  Demux3/5 -> Mux15/2
  Demux3/6 -> Mux15/3
  Mux14/1 -> Mux16/1
  Demux3/7 -> Mux16/2
  Mux15/1 -> Mux17/1
  Demux3/8 -> Mux17/2
  Mux16/1 -> Multiport Switch2/2
  Mux17/1 -> Multiport Switch2/3
  region 4/1 -> Demux4/1
  Demux4/1 -> Mux22/1
  Demux4/2 -> Mux22/2
  Demux4/3 -> Mux22/3
  Demux4/4 -> Mux23/1
  Demux4/5 -> Mux23/2
  Demux4/6 -> Mux23/3
  Demux4/7 -> Mux24/1
  Demux4/8 -> Mux24/2
  Demux4/9 -> Mux24/3
  Demux4/10 -> Mux25/1
  Demux4/11 -> Mux25/2
  Demux4/12 -> Mux25/3
  Mux22/1 -> Mux18/1
  Demux4/13 -> Mux18/2
  Mux23/1 -> Mux19/1
  Demux4/14 -> Mux19/2
  Mux24/1 -> Mux20/1
  Demux4/15 -> Mux20/2
  Mux25/1 -> Mux21/1
  Demux4/16 -> Mux21/2
  Mux18/1 -> Multiport Switch4/2
  Mux20/1 -> Multiport Switch4/4
  Mux21/1 -> Multiport Switch4/5
  Mux19/1 -> Multiport Switch4/3
  Constant6/1 -> Multiport Switch3/4, Multiport Switch4/6, Multiport Switch2/4, Multiport Switch1/6

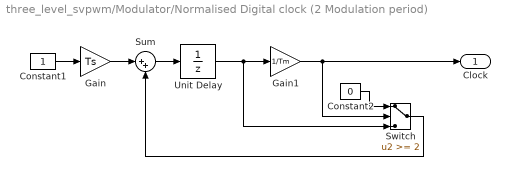
== system three_level_svpwm/Modulator/Normalised Digital clock (2 Modulation period) ==
  Constant1 : Constant
  Constant2 : Constant  Value=0
  Gain : Gain  Gain=Ts
  Gain1 : Gain  Gain=1/Tm
  Sum : Sum  Inputs=|++
  Switch : Switch  Threshold=2
  Unit Delay : UnitDelay  SampleTime=Ts
  Clock : Outport
  wires:
  Unit Delay/1 -> Switch/3, Gain1/1
  Gain/1 -> Sum/1
  Gain1/1 -> Clock/1, Switch/2
  Constant2/1 -> Switch/1
  Sum/1 -> Unit Delay/1
  Constant1/1 -> Gain/1
  Switch/1 -> Sum/2

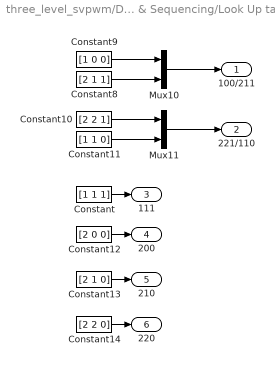
== system three_level_svpwm/Duty Cycle Calculation Short Vector Selection & Sequencing/Look Up table Switching sequence for different regions/First Sextant Switching Vector Look-Up Table ==
  Constant : Constant  Value=[1 1 1]
  Constant10 : Constant  Value=[2 2 1]
  Constant11 : Constant  Value=[1 1 0]
  Constant12 : Constant  Value=[2 0 0]
  Constant13 : Constant  Value=[2 1 0]
  Constant14 : Constant  Value=[2 2 0]
  Constant8 : Constant  Value=[2 1 1]
  Constant9 : Constant  Value=[1 0 0]
  Mux10 : Mux  Inputs=2
  Mux11 : Mux  Inputs=2
  100/211 : Outport
  221/110 : Outport  Port=2
  111 : Outport  Port=3
  200 : Outport  Port=4
  210 : Outport  Port=5
  220 : Outport  Port=6
  wires:
  Constant8/1 -> Mux10/2
  Constant10/1 -> Mux11/1
  Constant11/1 -> Mux11/2
  Mux11/1 -> 221/110/1
  Mux10/1 -> 100/211/1
  Constant9/1 -> Mux10/1
  Constant/1 -> 111/1
  Constant14/1 -> 220/1
  Constant12/1 -> 200/1
  Constant13/1 -> 210/1
